simulink model "simulacao_tanque"  (R2018a)
settings: Solver=VariableStepAuto  StartTime=0.0  StopTime=14000  RelTol=1e-3
values from neighbouring files (symbols this model uses):
  A =     [modelos.mat]    (also in termos_de_Ad.m = double(subs(jacobian([f1;f2],[h4 h3]),[h4 h3 u],[sp_h4 sp_h3)
  B =     [modelos.mat]    (also in termos_de_Ad.m = double(subs(jacobian([f1;f2],u),u,sp_u)))
  C =     [modelos.mat]    (also in termos_de_Ad.m = [0 1]; validacao_tanques.m = [0 1])
  D =     [modelos.mat]    (also in termos_de_Ad.m = 0; validacao_tanques.m = 0)
  sp_h3 = 0.48    [modelos.mat]    (also in termos_de_Ad.m = sp_h3*1e-2; validacao_tanques.m)
settings Model: Creator=tarsi  LastModifiedBy=tarsi

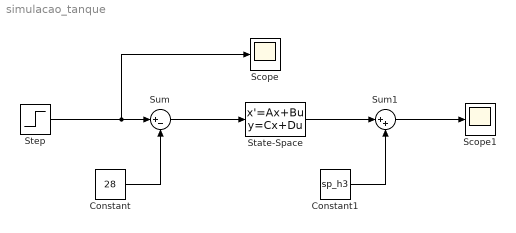
== system simulacao_tanque ==
  Constant : Constant  Value=28
  Constant1 : Constant  Value=sp_h3
  Scope : Scope
  Scope1 : Scope
  State-Space : StateSpace  A=A  B=B  C=C  D=D  InitialCondition=0
  Step : Step  Time=7000  Before=26  After=30  SampleTime=0
  Sum : Sum  Inputs=|+-
  Sum1 : Sum  Inputs=|++
  wires:
  Sum/1 -> State-Space/1
  State-Space/1 -> Sum1/1
  Constant/1 -> Sum/2
  Constant1/1 -> Sum1/2
  Step/1 -> Scope/1, Sum/1
  Sum1/1 -> Scope1/1
